simulink model "simulation_gripen_lqg_trajectory_following"  (R2024b)
settings: Solver=ode15s  StartTime=0.0  StopTime=500  RelTol=1e-3  EnableMultiTasking=on
undefined symbols (not defined in the file): A, A_kf, B, B_kf, C, C_kf, D, D_kf, Klq_eta, Klq_x, theta_dot, x0
libraries: simulink x1
settings Model: Creator=scattolini  LastModifiedBy=Davvy
settings SolverCC: AlgebraicLoopSolver=TrustRegion
settings DataIOCC: LimitDataPoints=on  SaveFormat=Array  SignalLoggingSaveFormat=ModelDataLogs  ReturnWorkspaceOutputs=off
settings OptimizationCC: ExpressionDepthLimit=2147483647  InitFltsAndDblsToZero=on  LifeSpan=inf
settings DebuggingCC: SaveWithParameterizedLinksMsg=none  UnderspecifiedInitializationDetection=Classic  MergeDetectMultiDrivingBlocksExec=none  SignalResolutionControl=TryResolveAllWithWarning  SolverPrmCheckMsg=warning  MultiTaskDSMMsg=warning  MultiTaskCondExecSysMsg=none  FcnCallInpInsideContextMsg=warning  UnconnectedInputMsg=warning  UnconnectedOutputMsg=warning  UnconnectedLineMsg=warning  StateNameClashWarn=warning  SFUnexpectedBacktrackingDiag=warning  SFNoUnconditionalDefaultTransitionDiag=warning  SFExecutionAtInitializationDiag=none  ArithmeticOperatorsInVariantConditions=warning
settings HardwareCC: ProdBitPerPointer=32  ProdBitPerSizeT=32  ProdBitPerPtrDiffT=32  ProdLargestAtomicFloat=None  ProdIntDivRoundTo=Undefined  ProdEndianess=Unspecified  ProdWordSize=32  ProdHWDeviceType=32-bit Generic
settings ModelReferenceCC: EnableRefExpFcnMdlSchedulingChecks=on  PropagateSignalLabelsOutOfModel=off
settings SFSimCC: SimUseLocalCustomCode=off  CustomCodeUndefinedFunction=UseInterfaceOnly
settings RTWCC: RTWUseLocalCustomCode=off  GPUComputeCapability=3.5  DLArmComputeVersion=19.05
settings CodeAppCC: StateflowObjectComments=on
settings GRTTargetCC: TargetFcnLib=ansi_tfl_tmw.mat  TargetLangStandard=C89/C90 (ANSI)  CombineOutputUpdateFcns=off  GRTInterface=on
settings ConfigComp: CovMetricSettings=dw  CovSaveCumulativeToWorkspaceVar=on  CovSaveSingleToWorkspaceVar=on  CovExternalEMLEnable=off

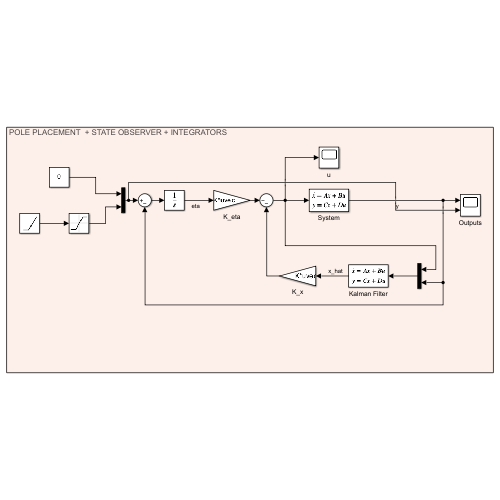
[thumbnail: Simulink's stored preview of the top-level diagram]
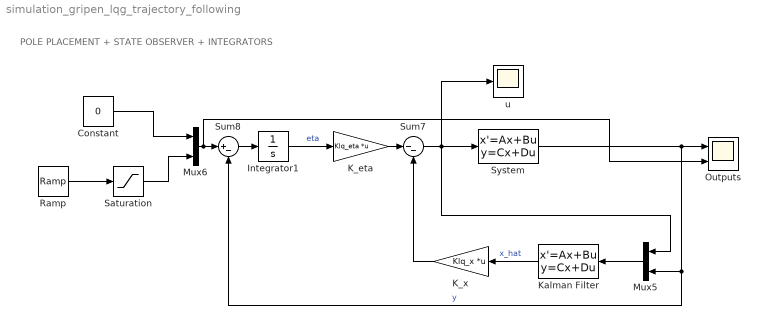
== system simulation_gripen_lqg_trajectory_following ==
  note: POLE PLACEMENT + STATE OBSERVER + INTEGRATORS
  Constant : Constant  Value=0
  Integrator1 : Integrator
  K_eta : Gain  Gain=Klq_eta  Multiplication=Matrix(K*u) (u vector)
  K_x : Gain  Gain=Klq_x  Multiplication=Matrix(K*u) (u vector)
  Kalman Filter : StateSpace  A=A_kf  B=B_kf  C=C_kf  D=D_kf  InitialCondition=0
  Mux5 : Mux  Inputs=2
  Mux6 : Mux  Inputs=2
  Outputs : Scope  NumInputPorts=2
  Ramp : simulink/Sources/Ramp  slope=theta_dot  start=100  InitialOutput=0
  Saturation : Saturate  UpperLimit=pi/2  LowerLimit=0
  Sum7 : Sum  Inputs=|--
  Sum8 : Sum  Inputs=|+-
  System : StateSpace  A=A  B=B  C=C  D=D  InitialCondition=x0
  u : Scope
  wires:
  K_x/1 -> Sum7/2
  Mux5/1 -> Kalman Filter/1
  System/1 -> Outputs/1, Mux5/2, Sum8/2  "y"
  Kalman Filter/1 -> K_x/1  "x_hat"
  K_eta/1 -> Sum7/1
  Sum7/1 -> u/1, Mux5/1, System/1
  Integrator1/1 -> K_eta/1  "eta"
  Sum8/1 -> Integrator1/1
  Mux6/1 -> Outputs/2, Sum8/1
  Constant/1 -> Mux6/1
  Saturation/1 -> Mux6/2
  Ramp/1 -> Saturation/1
